simulink model "Const2b_export"  (Simulink 7.9)
settings: Solver=ode45  StartTime=0.0  StopTime=10.0  RelTol=1e-3
settings Model: Creator=boakes  LastModifiedBy=boakes

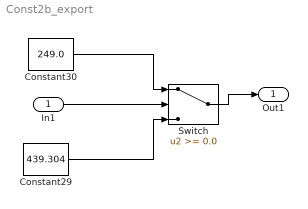
== system Const2b_export ==
  In1 : Inport
  Constant29 : Constant  Value=439.304
  Constant30 : Constant  Value=249.0
  Switch : Switch  Threshold=0.0
  Out1 : Outport
  wires:
  Constant29/1 -> Switch/3
  In1/1 -> Switch/2
  Switch/1 -> Out1/1
  Constant30/1 -> Switch/1
